simulink model "exnb4137986_Q3"  (R2023b)
settings: Solver=FixedStepAuto  StartTime=0  StopTime=100  FixedStep=0.01  RelTol=1e-3
settings Model: Creator=therk  LastModifiedBy=therk

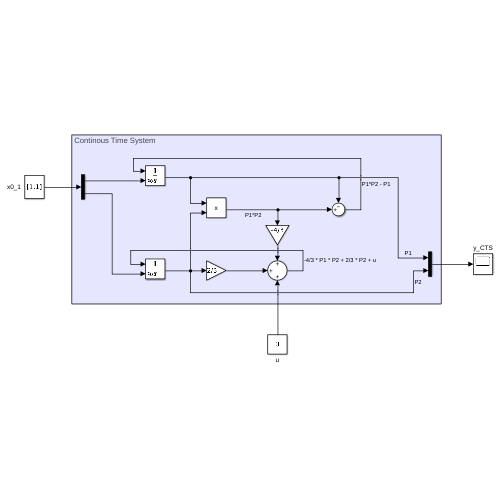
[thumbnail: Simulink's stored preview of the top-level diagram]
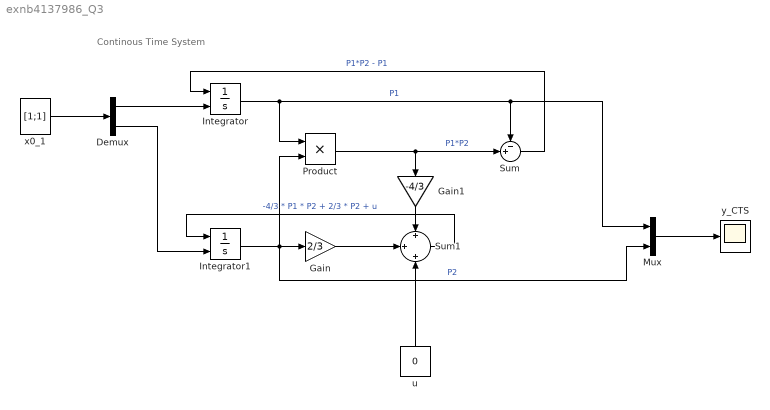
== system exnb4137986_Q3 ==
  note: Continous Time System
  Demux : Demux  Outputs=2
  Gain : Gain  Gain=2/3
  Gain1 : Gain  Gain=-4/3
  Integrator : Integrator  InitialConditionSource=external
  Integrator1 : Integrator  InitialConditionSource=external
  Mux : Mux  Inputs=2
  Product : Product
  Sum : Sum  Inputs=-+|
  Sum1 : Sum  Inputs=+|+|+
  u : Constant  Value=0
  x0_1 : Constant  Value=[1;1]
  y_CTS : Scope
  wires:
  Mux/1 -> y_CTS/1
  Demux/1 -> Integrator/2
  Demux/2 -> Integrator1/2
  Integrator1/1 -> Gain/1, Mux/2, Product/2  "P2"
  Integrator/1 -> Mux/1, Sum/1, Product/1  "P1"
  x0_1/1 -> Demux/1
  Product/1 -> Sum/2, Gain1/1  "P1*P2"
  Sum1/1 -> Integrator1/1  "-4/3 * P1 * P2 + 2/3 * P2 + u"
  Sum/1 -> Integrator/1  "P1*P2 - P1"
  u/1 -> Sum1/3
  Gain/1 -> Sum1/2
  Gain1/1 -> Sum1/1
